simulink model "fuelcell"  (R2017a)
settings: Solver=VariableStepAuto  StartTime=0.0  StopTime=10.0  RelTol=1e-3
libraries: fl_lib x7, nesl_utility x5
settings Model: Creator=mcall  LastModifiedBy=mcall

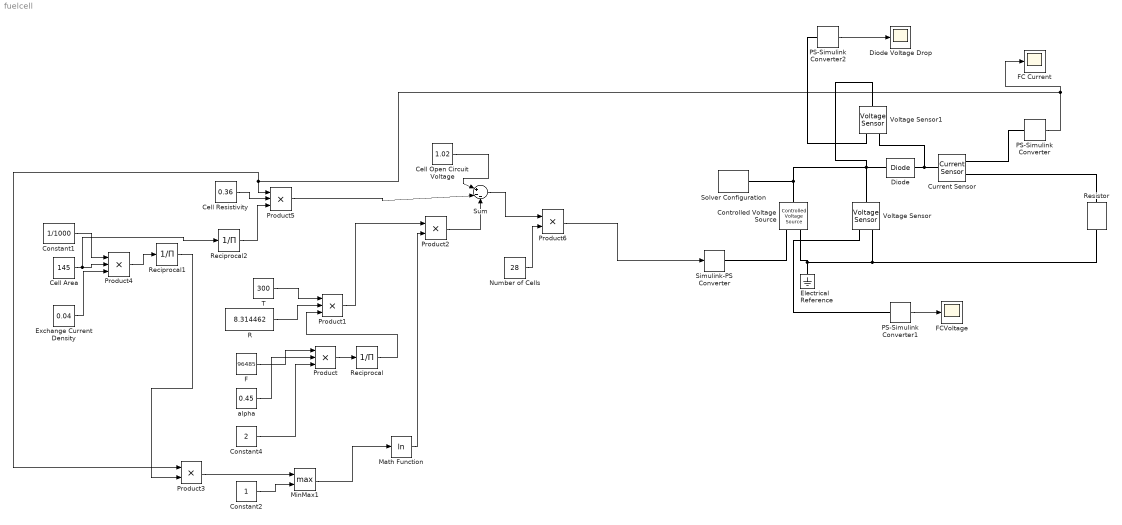
== system fuelcell ==
  Cell Area : Constant  Value=145
  Cell Open Circuit Voltage : Constant  Value=1.02
  Cell Resistivity : Constant  Value=0.36
  Constant1 : Constant  Value=1/1000
  Constant2 : Constant
  Constant4 : Constant  Value=2
  Controlled Voltage Source : fl_lib/Electrical/Electrical Sources/Controlled Voltage Source
  Current Sensor : fl_lib/Electrical/Electrical Sensors/Current Sensor
  Diode : fl_lib/Electrical/Electrical Elements/Diode  Vf=0.6 V  Ron=0.3 Ohm  Goff=1e-8 1/Ohm  i_specify=off  i_priority=None  i=0 A  i_nominal_specify=off  i_nominal_unit=A  i_nominal_value=1  v_specify=off  v_priority=None  v=0 V  v_nominal_specify=off  v_nominal_unit=V  v_nominal_value=1
  Diode Voltage Drop : Scope
  Electrical Reference : fl_lib/Electrical/Electrical Elements/Electrical Reference
  Exchange Current Density : Constant  Value=0.04
  F : Constant  Value=96485
  FC Current : Scope
  FCVoltage : Scope
  Math Function : Math  Operator=log  SaturateOnIntegerOverflow=on
  MinMax1 : MinMax  Function=max  Inputs=2
  Number of Cells : Constant  Value=28
  PS-Simulink Converter : nesl_utility/PS-Simulink Converter  PhysicalDomain=network_engine_domain  SubClassName=ps_output  LeftPortType=input  RightPortType=output  PseudoPeriodic=off  Frequencies=[]  Unit=1  AffineConversion=off
  PS-Simulink Converter1 : nesl_utility/PS-Simulink Converter  PhysicalDomain=network_engine_domain  SubClassName=ps_output  LeftPortType=input  RightPortType=output  PseudoPeriodic=off  Frequencies=[]  Unit=1  AffineConversion=off
  PS-Simulink Converter2 : nesl_utility/PS-Simulink Converter  PhysicalDomain=network_engine_domain  SubClassName=ps_output  LeftPortType=input  RightPortType=output  PseudoPeriodic=off  Frequencies=[]  Unit=1  AffineConversion=off
  Product{,1,4..5} (4 alike) : Product  Inputs=3
  Product2 : Product
  Product3 : Product
  Product6 : Product
  R : Constant  Value=8.314462
  Reciprocal : Product  Inputs=/  SaturateOnIntegerOverflow=on  RndMeth=Zero
  Reciprocal1 : Product  Inputs=/  SaturateOnIntegerOverflow=on  RndMeth=Zero
  Reciprocal2 : Product  Inputs=/  SaturateOnIntegerOverflow=on  RndMeth=Zero
  Resistor : fl_lib/Electrical/Electrical Elements/Resistor  R=1 Ohm  i_specify=off  i_priority=None  i=0 A  i_nominal_specify=off  i_nominal_unit=A  i_nominal_value=1  v_specify=off  v_priority=None  v=0 V  v_nominal_specify=off  v_nominal_unit=V  v_nominal_value=1
  Simulink-PS Converter : nesl_utility/Simulink-PS Converter  PhysicalDomain=network_engine_domain  SubClassName=ps_input  LeftPortType=input  RightPortType=output  PseudoPeriodic=off  Frequencies=[]  NoiseDistribution=none  NoiseParameters=[]  Unit=1  AffineConversion=off  FilteringAndDerivatives=provide  SimscapeFilterOrder=1  InputFilterTimeConstant=0.001  UdotUserProvided=0
  Solver Configuration : nesl_utility/Solver Configuration  PhysicalDomain=network_engine_domain  SubClassName=solver  LeftPortType=input  RightPortType=generic  Accelerate=off  Tones=[]  Harmonics=[]  SimulateNoise=off  Profile=off  UseLocalSampling=off  EnableSwitchedLinearOptims=on  FrequencyDomain=off  UseCCode=off  RelTol=0.001  AbsTol=1e-06  MinStep=1e-09  ToWorkspace=off  RevertToSquareIcSolve=off  NumHomotopyIterations=100  PhasorMode=off  PhasorModeNumHarmonics=1  OverrideAbsTol=off  DoDC=off  ResidualTolerance=1e-09  UseLocalSolver=off  LocalSolverChoice=NE_BACKWARD_EULER_ADVANCER  LocalSolverSampleTime=0.001  DoFixedCost=off  MaxNonlinIter=3  MaxModeIter=2  LinearAlgebra=Sparse  DelaysMemoryBudget=1024  AutomaticFiltering=on  FilteringTimeConstant=0.001
  Sum : Sum  Inputs=|+--
  T : Constant  Value=300
  Voltage Sensor : fl_lib/Electrical/Electrical Sensors/Voltage Sensor
  Voltage Sensor1 : fl_lib/Electrical/Electrical Sensors/Voltage Sensor
  alpha : Constant  Value=0.45
  wires:
  PS-Simulink Converter2/1 -> Diode Voltage Drop/1
  Product6/1 -> Simulink-PS Converter/1
  Product3/1 -> MinMax1/1
  R/1 -> Product1/2
  Reciprocal/1 -> Product1/3
  MinMax1/1 -> Math Function/1
  Cell Area/1 -> Reciprocal2/1, Product4/2
  alpha/1 -> Product/2
  PS-Simulink Converter1/1 -> FCVoltage/1
  PS-Simulink Converter/1 -> FC Current/1, Product3/1, Product5/1
  Reciprocal2/1 -> Product5/3
  Reciprocal1/1 -> Product3/2
  F/1 -> Product/1
  Product4/1 -> Reciprocal1/1
  Constant4/1 -> Product/3
  Cell Resistivity/1 -> Product5/2
  Constant1/1 -> Product4/1
  Product/1 -> Reciprocal/1
  Number of Cells/1 -> Product6/2
  Cell Open Circuit Voltage/1 -> Sum/1
  T/1 -> Product1/1
  Math Function/1 -> Product2/2
  Product1/1 -> Product2/1
  Sum/1 -> Product6/1
  Exchange Current Density/1 -> Product4/3
  Product5/1 -> Sum/2
  Product2/1 -> Sum/3
  Constant2/1 -> MinMax1/2
  connections:
  Diode/RConn1 -- Current Sensor/LConn1 -- Voltage Sensor1/RConn2
  Voltage Sensor/LConn1 -- Diode/LConn1 -- Voltage Sensor1/LConn1 -- Solver Configuration/RConn1 -- Controlled Voltage Source/LConn1
  Voltage Sensor/RConn2 -- Resistor/RConn1 -- Electrical Reference/LConn1 -- Controlled Voltage Source/RConn2
  Resistor/LConn1 -- Current Sensor/RConn2
  Simulink-PS Converter/RConn1 -- Controlled Voltage Source/RConn1
  Voltage Sensor/RConn1 -- PS-Simulink Converter1/LConn1
  Voltage Sensor1/RConn1 -- PS-Simulink Converter2/LConn1
  Current Sensor/RConn1 -- PS-Simulink Converter/LConn1
